simulink model "SimulinkComVies"  (R2013b)
settings: Solver=ode3  StartTime=0.0  StopTime=20  RelTol=1e-3
values from neighbouring files (symbols this model uses):
  Ad = 1    [inicializa.m]
  Ad_K = [1 -T ... (first row only)    [inicializa.m]
  Bd = T    (= 0.01)    [inicializa.m]
  Bd_K = [ T ... (first row only)    [inicializa.m]
  Bd_n = [T      0 ... (first row only)    [inicializa.m]
settings Model: Creator=ThiagoCordeiro  LastModifiedBy=ThiagoFelippe

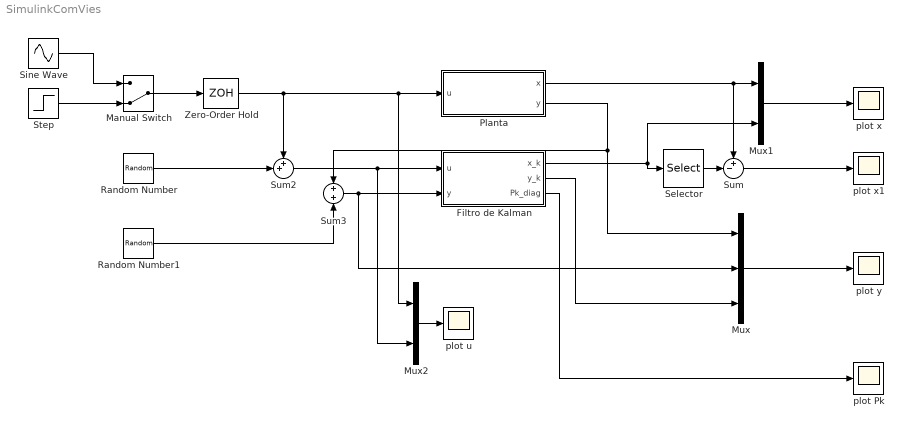
== system SimulinkComVies ==
  Filtro de Kalman : Subsystem
  Manual Switch : ManualSwitch  CurrentSetting=0
  Mux : Mux  Inputs=3
  Mux1 : Mux  Inputs=2
  Mux2 : Mux  Inputs=2
  Planta : Subsystem
  Random Number : RandomNumber  Mean=0.5  Seed=round(rand(1)*(2^32-1))  SampleTime=0.01
  Random Number1 : RandomNumber  Mean=[0; 0]  Variance=[1; 1]  Seed=round(rand(2,1)*(2^32-1))  SampleTime=0.01
  Selector : Selector  InputPortWidth=2  IndexOptions=Index vector (dialog)  Indices=[1]  OutputSizes=1
  Sine Wave : Sin  Amplitude=2  Phase=pi/2  SampleTime=0
  Step : Step  Time=0  After=2*pi/10  SampleTime=0
  Sum : Sum  Inputs=+-|
  Sum2 : Sum  Inputs=++|
  Sum3 : Sum  Inputs=+|+
  Zero-Order Hold : ZeroOrderHold  SampleTime=0.01
  plot Pk : Scope
      settings: ShowLegends=on  SaveName=ScopeData4
  plot u : Scope
      settings: ShowLegends=on  SaveName=ScopeData6
  plot x : Scope
  plot x1 : Scope
  plot y : Scope
      settings: ShowLegends=on  SaveName=ScopeData2
  wires:
  Mux/1 -> plot y/1
  Zero-Order Hold/1 -> Mux2/1, Planta/1(u), Sum2/1
  Random Number/1 -> Sum2/2
  Random Number1/1 -> Sum3/2
  Sum2/1 -> Mux2/2, Filtro de Kalman/1(u)
  Sum3/1 -> Mux/2, Filtro de Kalman/2(y)
  Planta/2(y) -> Mux/1, Sum3/1
  Planta/1(x) -> Sum/1, Mux1/1
  Filtro de Kalman/1(x_k) -> Selector/1, Mux1/2
  Mux1/1 -> plot x/1
  Filtro de Kalman/2(y_k) -> Mux/3
  Sum/1 -> plot x1/1
  Manual Switch/1 -> Zero-Order Hold/1
  Sine Wave/1 -> Manual Switch/1
  Step/1 -> Manual Switch/2
  Selector/1 -> Sum/2
  Filtro de Kalman/3(Pk_diag) -> plot Pk/1
  Mux2/1 -> plot u/1

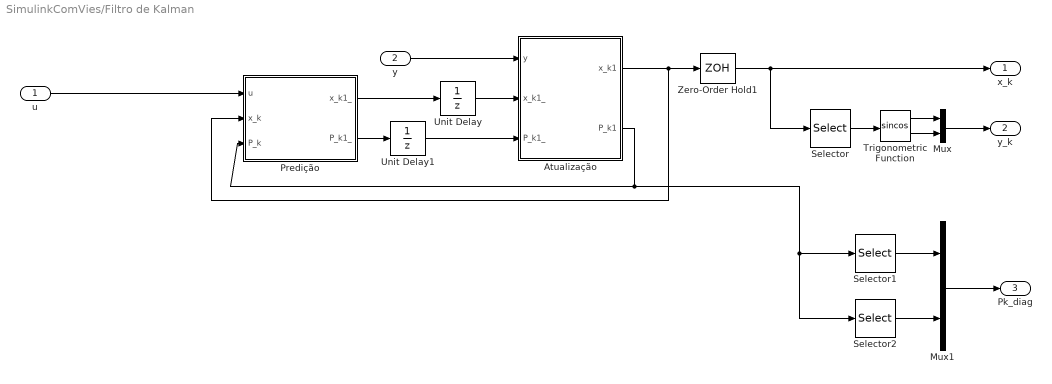
== system SimulinkComVies/Filtro de Kalman ==
  u : Inport
  y : Inport  Port=2
  Atualização : Subsystem
  Mux : Mux  Inputs=2
  Mux1 : Mux  Inputs=2
  Predição : Subsystem
  Selector : Selector  InputPortWidth=2  IndexOptions=Index vector (dialog)  Indices=[1]  OutputSizes=1
  Selector1 : Selector  NumberOfDimensions=2  InputPortWidth=2  IndexOptions=Index vector (dialog),Index vector (dialog)  Indices=[1],1  OutputSizes=1,1
  Selector2 : Selector  NumberOfDimensions=2  InputPortWidth=2  IndexOptions=Index vector (dialog),Index vector (dialog)  Indices=2,2  OutputSizes=1,1
  Trigonometric Function : Trigonometry  Operator=sincos
  Unit Delay : UnitDelay  InitialCondition=randn(2,1)  SampleTime=0.01
  Unit Delay1 : UnitDelay  InitialCondition=eye(2)  SampleTime=0.01
  Zero-Order Hold1 : ZeroOrderHold  SampleTime=0.01
  x_k : Outport
  y_k : Outport  Port=2
  Pk_diag : Outport  Port=3
  wires:
  u/1 -> Predição/1(u)
  y/1 -> Atualização/1(y)
  Atualização/1(x_k1) -> Predição/2(x_k), Zero-Order Hold1/1
  Atualização/2(P_k1) -> Selector1/1, Selector2/1, Predição/3(P_k)
  Predição/2(P_k1_) -> Unit Delay1/1
  Unit Delay1/1 -> Atualização/3(P_k1_)
  Unit Delay/1 -> Atualização/2(x_k1_)
  Predição/1(x_k1_) -> Unit Delay/1
  Mux/1 -> y_k/1
  Trigonometric Function/1 -> Mux/1
  Trigonometric Function/2 -> Mux/2
  Selector/1 -> Trigonometric Function/1
  Zero-Order Hold1/1 -> Selector/1, x_k/1
  Selector1/1 -> Mux1/1
  Selector2/1 -> Mux1/2
  Mux1/1 -> Pk_diag/1

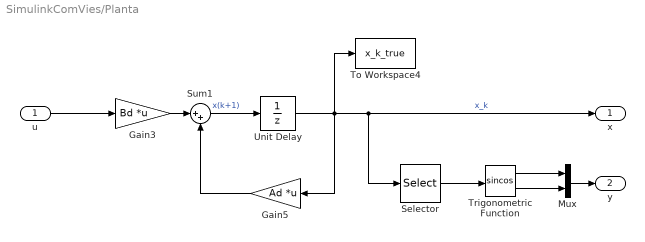
== system SimulinkComVies/Planta ==
  u : Inport
  Gain3 : Gain  Gain=Bd  Multiplication=Matrix(K*u)
  Gain5 : Gain  Gain=Ad  Multiplication=Matrix(K*u)
  Mux : Mux  Inputs=2
  Selector : Selector  InputPortWidth=2  IndexOptions=Index vector (dialog)  Indices=[1]  OutputSizes=1
  Sum1 : Sum  Inputs=|++
  To Workspace4 : ToWorkspace  VariableName=x_k_true  SampleTime=-1  SaveFormat=Timeseries
  Trigonometric Function : Trigonometry  Operator=sincos
  Unit Delay : UnitDelay  InitialCondition=[0]  SampleTime=-1
  x : Outport
  y : Outport  Port=2
  wires:
  Gain3/1 -> Sum1/1
  Sum1/1 -> Unit Delay/1  "x(k+1)"
  Unit Delay/1 -> Selector/1, x/1, To Workspace4/1, Gain5/1  "x_k"
  Gain5/1 -> Sum1/2
  u/1 -> Gain3/1
  Trigonometric Function/1 -> Mux/1
  Trigonometric Function/2 -> Mux/2
  Mux/1 -> y/1
  Selector/1 -> Trigonometric Function/1

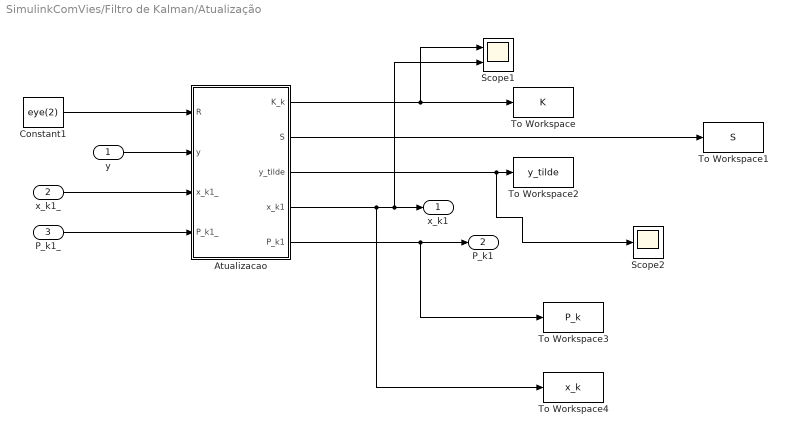
== system SimulinkComVies/Filtro de Kalman/Atualização ==
  y : Inport
  x_k1_ : Inport  Port=2
  P_k1_ : Inport  Port=3
  Atualizacao : MATLAB Function  TreatAsAtomicUnit=on  SystemSampleTime=0.01
  Constant1 : Constant  Value=eye(2)
  Scope1 : Scope  NumInputPorts=2
      settings: YMin=-5~-5  YMax=5~5  SaveName=ScopeData3
  Scope2 : Scope
      settings: SaveName=ScopeData5
  To Workspace : ToWorkspace  VariableName=K  SampleTime=-1  SaveFormat=Timeseries
  To Workspace1 : ToWorkspace  VariableName=S  SampleTime=-1  SaveFormat=Timeseries
  To Workspace2 : ToWorkspace  VariableName=y_tilde  SampleTime=-1  SaveFormat=Timeseries
  To Workspace3 : ToWorkspace  VariableName=P_k  SampleTime=-1  SaveFormat=Timeseries
  To Workspace4 : ToWorkspace  VariableName=x_k  SampleTime=-1  SaveFormat=Timeseries
  x_k1 : Outport
  P_k1 : Outport  Port=2
  wires:
  y/1 -> Atualizacao/2(y)
  x_k1_/1 -> Atualizacao/3(x_k1_)
  P_k1_/1 -> Atualizacao/4(P_k1_)
  Atualizacao/4(x_k1) -> To Workspace4/1, Scope1/2, x_k1/1
  Atualizacao/5(P_k1) -> To Workspace3/1, P_k1/1
  Constant1/1 -> Atualizacao/1(R)
  Atualizacao/1(K_k) -> Scope1/1, To Workspace/1
  Atualizacao/2(S) -> To Workspace1/1
  Atualizacao/3(y_tilde) -> Scope2/1, To Workspace2/1

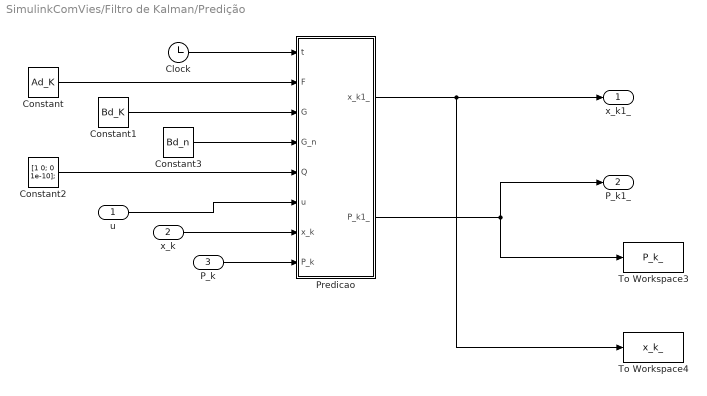
== system SimulinkComVies/Filtro de Kalman/Predição ==
  u : Inport
  x_k : Inport  Port=2
  P_k : Inport  Port=3
  Clock : Clock
  Constant : Constant  Value=Ad_K
  Constant1 : Constant  Value=Bd_K  VectorParams1D=off
  Constant2 : Constant  Value=[1 0; 0 1e-10];
  Constant3 : Constant  Value=Bd_n  VectorParams1D=off
  Predicao : MATLAB Function  TreatAsAtomicUnit=on  SystemSampleTime=0.01
  To Workspace3 : ToWorkspace  VariableName=P_k_  SampleTime=-1  SaveFormat=Timeseries
  To Workspace4 : ToWorkspace  VariableName=x_k_  SampleTime=-1  SaveFormat=Timeseries
  x_k1_ : Outport
  P_k1_ : Outport  Port=2
  wires:
  Predicao/1(x_k1_) -> To Workspace4/1, x_k1_/1
  Predicao/2(P_k1_) -> P_k1_/1, To Workspace3/1
  u/1 -> Predicao/6(u)
  x_k/1 -> Predicao/7(x_k)
  P_k/1 -> Predicao/8(P_k)
  Constant/1 -> Predicao/2(F)
  Constant1/1 -> Predicao/3(G)
  Constant2/1 -> Predicao/5(Q)
  Clock/1 -> Predicao/1(t)
  Constant3/1 -> Predicao/4(G_n)

== matlab function SimulinkComVies/Filtro de Kalman/Atualização/Atualizacao ==
  data: R input; K_k output; S output; y_tilde output; y input; x_k1_ input; P_k1_ input; x_k1 output; P_k1 output
function [K_k, S, y_tilde, x_k1, P_k1] = fcn(R, y, x_k1_, P_k1_)
%#codegen

y_hat = [ sin(x_k1_(1));
          cos(x_k1_(1))];
H =     [ cos(x_k1_(1))  0;
         -sin(x_k1_(1))  0];

S = H * P_k1_ * H' + R;
Pxy = P_k1_ * H';
K_k  =  Pxy / S;
KH = K_k*H;
I = eye(size(KH));
I_KH = I - KH;
P_k1 = I_KH * P_k1_ * I_KH' + K_k * R * K_k';


y_tilde = y - y_hat;
x_k1 = x_k1_ + K_k * y_tilde;

== matlab function SimulinkComVies/Filtro de Kalman/Predição/Predicao ==
  data: t input; F input; G input; G_n input; Q input; u input; x_k1_ output; x_k input; P_k input; P_k1_ output
function [x_k1_,P_k1_] = fcn(t, F, G, G_n, Q, u, x_k, P_k)
%#codegen
if t >= 0
    x_k1_ = F*x_k + G*u;
    P_k1_ = F*P_k*F' + G_n*Q*G_n';
else
    x_k1_ = x_k;
    P_k1_ = P_k;
end
